simulink model "InterModel_RX"  (Simulink 7.4)
settings: Solver=FixedStepDiscrete  SolverMode=SingleTasking  StartTime=0.0  StopTime=inf  FixedStep=.02  RelTol=1e-3
settings Model: Creator=fwornle  LastModifiedBy=fw  ExtModeTrigDuration=500
settings ConfigSet: Description=rtmc9s12target_R2008a
settings DataIOCC: SignalLoggingName=sigsOut
settings OptimizationCC: BooleanDataType=off  InitFltsAndDblsToZero=on
settings DebuggingCC: SaveWithParameterizedLinksMsg=none  SignalResolutionControl=TryResolveAllWithWarning  SolverPrmCheckMsg=none  MultiTaskDSMMsg=warning  MultiTaskCondExecSysMsg=none  StrictBusMsg=None
settings HardwareCC: ProdBitPerInt=16  ProdEndianess=BigEndian  ProdWordSize=16  ProdHWDeviceType=Motorola HC12  TargetHWDeviceType=32-bit Generic  ProdEqTarget=off
settings RTWCC: GenerateMakefile=off  TemplateMakefile=grt_msvc.tmf  Description="Visual C/C++ Project Makefile only for the \"grt\" target"  ProcessScript=grt_make_rtw_hook  IncludeERTFirstTime=on
settings GRTTargetCC: TargetFcnLib=ansi_tfl_tmw.mat

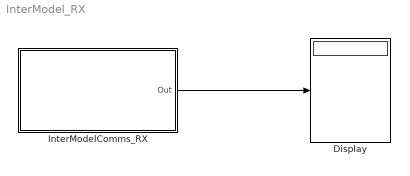
== system InterModel_RX ==
  Display : Display
  InterModelComms_RX : Subsystem  Tag=mcTarget_freePortCommsTX  mask{sampletime=0.1, channel=0, buf_size=5, data_type=UINT8}
      mask prompts: sampletime "Sample time"; channel "Channel number"; buf_size "Number of elements"; data_type "Data Type"
      mask init:
      | [buf_sizestr, channelstr, data_type_str, sampletime_str] = mbc_intermodelrxd(sampletime, channel, buf_size, data_type);
      mask Help: web('freePortComms_txd.html');
      mask StyleString: edit,edit,edit,popup(SINGLE|INT8|UINT8|INT16|UINT16|INT32|UINT32|BOOLEAN)
      mask Display: fprintf('Receive %s element(s)\nChannel: %s\nData type: %s\n Sample rate: %s', buf_sizestr, channelstr, data_type_str, sampletime_str)
  wires:
  InterModelComms_RX/1(Out) -> Display/1

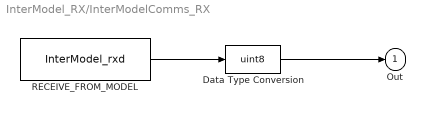
== system InterModel_RX/InterModelComms_RX ==
  Data Type Conversion : DataTypeConversion  OutDataTypeMode=uint8  OutDataType=sfix(16)  OutScaling=2^0  OutDataTypeStr=uint8  SaturateOnIntegerOverflow=on  RndMeth=Zero
  RECEIVE_FROM_MODEL : S-Function  Tag=mcTarget_freePortCommsTX  FunctionName=InterModel_rxd  Parameters=sampletime, channel, buf_size, data_type  EnableBusSupport=off
  Out : Outport  OutDataType=sfix(16)  OutScaling=2^0
  wires:
  RECEIVE_FROM_MODEL/1 -> Data Type Conversion/1
  Data Type Conversion/1 -> Out/1
